simulink model "sampleModel1612"  (R2023a)
settings: Solver=VariableStepAuto  StartTime=0.0  StopTime=10.0  RelTol=1e-3
libraries: hdlsllib x6, simulink x2
settings Model: Creator=user1  LastModifiedBy=user1

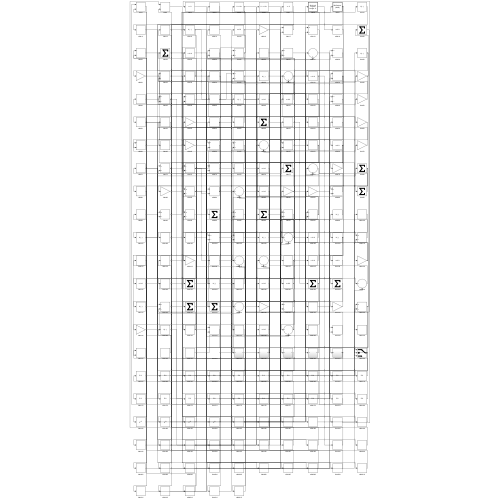
[thumbnail: Simulink's stored preview of the top-level diagram]
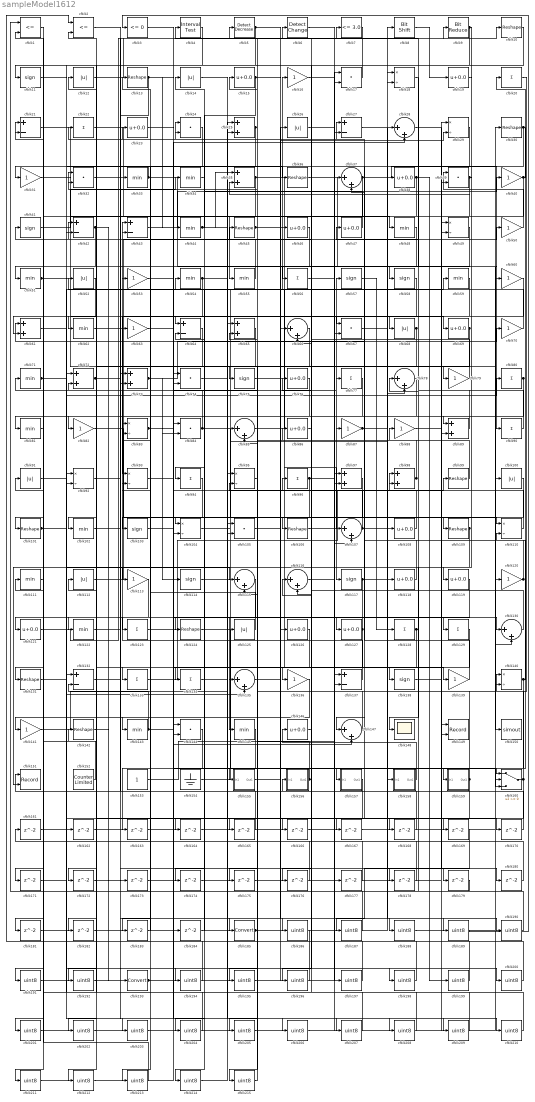
== system sampleModel1612 ==
  cfblk1 : RelationalOperator  Operator=<=  OutDataTypeStr=boolean  InputSameDT=off
  cfblk{10,13,30,36,45,99,101,106,109,124,131,142} (12 alike) : Reshape
  cfblk{12,14,26,52,68,91,100,112,125} (9 alike) : Abs  SaturateOnIntegerOverflow=off
  cfblk{33..34,44,48,51,54..55,59,62,71,81,102,111,122,143,145} (16 alike) : MinMax
  cfblk{11,41,57..58,75,103,114,117,138} (9 alike) : Signum
  cfblk{18,29,49,83,92..93,95,104,110,140} (10 alike) : Product  Inputs=*/  RndMeth=Zero  SaturateOnIntegerOverflow=on
  cfblk{17,24,32,39,67,74,84,105,144} (9 alike) : DotProduct  OutDataTypeStr=Inherit: Inherit via internal rule
  cfblk{28,37,66,78,85,107,115..116,130,135,147} (11 alike) : Sum  Inputs=|++
  cfblk{15,19,23,38,46..47,69,76,86,108,118..119,121,126..127,146} (16 alike) : Bias  Bias=0.0  SaturateOnIntegerOverflow=off
  cfblk{16,31,40,50,53,60,63,70,79,82,87..88,113,120,136,139,141} (17 alike) : Gain
  cfblk{20,22,56,77,80,90,94,96,123,128..129,133..134} (13 alike) : Sum  Inputs=+
  cfblk{21,27,42..43,64,132,137} (7 alike) : Sum  Inputs=+-
  cfblk148 : Scope
  cfblk149 : Record  FileSettingsInternal="{\"entries\":[{\"content\":{\"excelSettings\":{\"content\":{},\"type\":\"Streamout.ExcelSettings\"}},\"type\":\"Streamout.FileSettingStorage\",\"uuid\":\"\"}],\"packageUris\":[\"http:\\/\\/schema.mathworks.com\\/mf0\\/streamout_blocks\\/R2020a\"],\"version\":\"1.0\"}"  Layout=[1 1]  SignalsInternal="{\"entries\":[{\"content\":{\"signals\":[{\"content\":{\"blockPath\":[],\"dimensions\":[1],\"domain\":\"\",\"lineColor\":\"#a2142f\",\"plots\":[1],\"port\":1,\"signalID\":2323,\"signalName\":\"XY Graph:1\"},\"type\":\"RecordBlkView.Signal\",\"uuid\":\"\"},{\"content\":{\"blockPath\":[],\"dimensions\":[1],\"domain\":\"\",\"lineColor\":\"#139fff\",\"plots\":[1],\"port\":2,\"signalID\":2326,\"signalName\":\"XY Graph:2\"},\"type\":\"RecordBlkView.Signal\",\"uuid\":\"\"}]},\"type\":\"RecordBlkView.InputSignals\",\"uuid\":\"\"}],\"packageUris\":[\"http:\\/\\/schema.mathworks.com\\/mf0\\/streamout_blocks\\/R2020a\"],\"version\":\"1.0\"}"  VisualizationBindings="{\"xyplotplugin\":{\"info\":[{\"series\":[{\"bindingParametersList\":[{\"parameter\":\"X-Axis\",\"signalID\":2323,\"signalName\":\"XY Graph:1\"},{\"parameter\":\"Y-Axis\",\"signalID\":2326,\"signalName\":\"XY Graph:2\"}],\"seriesID\":49323}],\"subplotID\":1}]}}"  CompatibilityTag=XY  st=-1
  cfblk150 : ToWorkspace  VariableName=simout  SaveFormat=Timeseries  SampleTime=-1
  cfblk151 : Record  FileSettingsInternal="{\"entries\":[{\"content\":{\"excelSettings\":{\"content\":{},\"type\":\"Streamout.ExcelSettings\"}},\"type\":\"Streamout.FileSettingStorage\",\"uuid\":\"\"}],\"packageUris\":[\"http:\\/\\/schema.mathworks.com\\/mf0\\/streamout_blocks\\/R2020a\"],\"version\":\"1.0\"}"  Layout=[1 1]  SignalsInternal="{\"entries\":[{\"content\":{\"signals\":[{\"content\":{\"blockPath\":[],\"dimensions\":[1],\"domain\":\"\",\"lineColor\":\"#a2142f\",\"plots\":[1],\"port\":1,\"signalID\":2331,\"signalName\":\"XY Graph:1\"},\"type\":\"RecordBlkView.Signal\",\"uuid\":\"\"},{\"content\":{\"blockPath\":[],\"dimensions\":[1],\"domain\":\"\",\"lineColor\":\"#139fff\",\"plots\":[1],\"port\":2,\"signalID\":2334,\"signalName\":\"XY Graph:2\"},\"type\":\"RecordBlkView.Signal\",\"uuid\":\"\"}]},\"type\":\"RecordBlkView.InputSignals\",\"uuid\":\"\"}],\"packageUris\":[\"http:\\/\\/schema.mathworks.com\\/mf0\\/streamout_blocks\\/R2020a\"],\"version\":\"1.0\"}"  VisualizationBindings="{\"xyplotplugin\":{\"info\":[{\"series\":[{\"bindingParametersList\":[{\"parameter\":\"X-Axis\",\"signalID\":2331,\"signalName\":\"XY Graph:1\"},{\"parameter\":\"Y-Axis\",\"signalID\":2334,\"signalName\":\"XY Graph:2\"}],\"seriesID\":48579}],\"subplotID\":1}]}}"  CompatibilityTag=XY  st=-1
  cfblk152 : hdlsllib/Sources/Counter Limited  uplimit=7  tsamp=-1
  cfblk153 : Constant  SampleTime=-1
  cfblk154 : Ground
  cfblk155 : Subsystem
      settings: LibrarySourceBlock=|
      | hdlsllib/Ports &
      | Subsystems/Subsystem
  cfblk156 : Subsystem
      settings: LibrarySourceBlock=|
      | hdlsllib/Ports &
      | Subsystems/Subsystem
  cfblk157 : Subsystem
      settings: LibrarySourceBlock=|
      | hdlsllib/Ports &
      | Subsystems/Subsystem
  cfblk158 : Subsystem
      settings: LibrarySourceBlock=|
      | hdlsllib/Ports &
      | Subsystems/Subsystem
  cfblk159 : Subsystem
      settings: LibrarySourceBlock=|
      | hdlsllib/Ports &
      | Subsystems/Subsystem
  cfblk160 : Switch  SaturateOnIntegerOverflow=off  InputSameDT=off
  cfblk{161..184} (24 alike) : Delay  SampleTime=1
  cfblk185 : DataTypeConversion  SaturateOnIntegerOverflow=off  RndMeth=Floor
  cfblk{186..192,194..215} (29 alike) : DataTypeConversion  OutDataTypeStr=uint8  SaturateOnIntegerOverflow=off  RndMeth=Floor
  cfblk193 : DataTypeConversion  SaturateOnIntegerOverflow=off  RndMeth=Floor
  cfblk2 : RelationalOperator  Operator=<=  OutDataTypeStr=boolean  InputSameDT=off
  cfblk{25,35,61,65,72..73,89,97..98} (9 alike) : Sum
  cfblk3 : hdlsllib/Logic and Bit Operations/Compare To Zero  relop=<=  OutDataTypeStr=boolean
  cfblk4 : hdlsllib/Logic and Bit Operations/Interval Test  IntervalClosedRight=on  uplimit=0.5  IntervalClosedLeft=on  lowlimit=-0.5  OutDataTypeStr=boolean
  cfblk5 : simulink/Logic and Bit Operations/Detect Decrease  vinit=0.0  OutDataTypeStr=boolean
      settings: LibrarySourceBlock=|
      | hdlsllib/Logic and Bit
      | Operations/Detect
      | Decrease
  cfblk6 : simulink/Logic and Bit Operations/Detect Change  vinit=0  OutDataTypeStr=boolean
      settings: LibrarySourceBlock=|
      | hdlsllib/Logic and Bit
      | Operations/Detect
      | Change
  cfblk7 : hdlsllib/Logic and Bit Operations/Compare To Constant  relop=<=  const=3.0  OutDataTypeStr=boolean
  cfblk8 : hdlsllib/Logic and Bit Operations/Bit Shift  mode=Shift Left Logical  N=0
  cfblk9 : hdlsllib/Logic and Bit Operations/Bit Reduce  mode=AND
  wires:
  cfblk137/1 -> cfblk43/1
  cfblk57/1 -> cfblk128/1
  cfblk121/1 -> cfblk7/1
  cfblk5/1 -> cfblk42/2, cfblk178/1
  cfblk39/1 -> cfblk55/1, cfblk109/1, cfblk35/2
  cfblk112/1 -> cfblk45/1
  cfblk98/1 -> cfblk53/1, cfblk32/1
  cfblk114/1 -> cfblk16/1
  cfblk75/1 -> cfblk139/1
  cfblk37/1 -> cfblk90/1, cfblk66/2
  cfblk107/1 -> cfblk96/1, cfblk160/3
  cfblk130/1 -> cfblk41/1
  cfblk106/1 -> cfblk57/1
  cfblk62/1 -> cfblk25/1
  cfblk35/1 -> cfblk117/1, cfblk124/1
  cfblk113/1 -> cfblk121/1
  cfblk82/1 -> cfblk110/1
  cfblk31/1 -> cfblk68/1
  cfblk143/1 -> cfblk12/1, cfblk99/1
  cfblk158/1(Out1) -> cfblk146/1
  cfblk8/1 -> cfblk19/1
  cfblk36/1 -> cfblk120/1
  cfblk131/1 -> cfblk59/1
  cfblk99/1 -> cfblk78/1
  cfblk12/1 -> cfblk9/1
  cfblk51/1 -> cfblk150/1, cfblk191/1, cfblk194/1
  cfblk154/1 -> cfblk98/1
  cfblk33/1 -> cfblk158/1(In1), cfblk31/1
  cfblk10/1 -> cfblk56/1
  cfblk139/1 -> cfblk27/1
  cfblk64/1 -> cfblk93/1
  cfblk46/1 -> cfblk133/1
  cfblk1/1 -> cfblk51/1
  cfblk25/1 -> cfblk5/1, cfblk202/1
  cfblk125/1 -> cfblk13/1
  cfblk66/1 -> cfblk82/1
  cfblk84/1 -> cfblk106/1, cfblk72/2
  cfblk109/1 -> cfblk148/1, cfblk151/2
  cfblk53/1 -> cfblk155/1(In1)
  cfblk153/1 -> cfblk27/2
  cfblk73/1 -> cfblk70/1, cfblk84/2, cfblk28/2, cfblk138/1
  cfblk140/1 -> cfblk110/2, cfblk183/1
  cfblk118/1 -> cfblk61/1
  cfblk50/1 -> cfblk39/1
  cfblk9/1 -> cfblk119/1, cfblk92/2
  cfblk15/1 -> cfblk104/1, cfblk79/1
  cfblk38/1 -> cfblk176/1, cfblk199/1
  cfblk68/1 -> cfblk136/1, cfblk75/1
  cfblk11/1 -> cfblk36/1
  cfblk133/1 -> cfblk8/1
  cfblk22/1 -> cfblk118/1
  cfblk142/1 -> cfblk193/1
  cfblk56/1 -> cfblk137/2
  cfblk67/1 -> cfblk78/2
  cfblk2/1 -> cfblk185/1
  cfblk123/1 -> cfblk28/1
  cfblk42/1 -> cfblk101/1, cfblk173/1
  cfblk87/1 -> cfblk129/1, cfblk37/2
  cfblk117/1 -> cfblk127/1, cfblk160/2, cfblk181/1
  cfblk79/1 -> cfblk24/1
  cfblk104/1 -> cfblk18/1
  cfblk141/1 -> cfblk25/2
  cfblk41/1 -> cfblk34/1
  cfblk55/1 -> cfblk21/1
  cfblk111/1 -> cfblk131/1
  cfblk90/1 -> cfblk47/1
  cfblk135/1 -> cfblk46/1
  cfblk76/1 -> cfblk134/1
  cfblk136/1 -> cfblk141/1
  cfblk80/1 -> cfblk81/1, cfblk149/2
  cfblk100/1 -> cfblk147/1
  cfblk7/1 -> cfblk62/1
  cfblk44/1 -> cfblk24/2, cfblk67/1, cfblk35/1
  cfblk20/1 -> cfblk140/1
  cfblk24/1 -> cfblk123/1
  cfblk19/1 -> cfblk89/1
  cfblk43/1 -> cfblk40/1
  cfblk52/1 -> cfblk61/2
  cfblk58/1 -> cfblk83/1
  cfblk160/1 -> cfblk42/1, cfblk174/1, cfblk175/1
  cfblk23/1 -> cfblk130/1
  cfblk21/1 -> cfblk84/1
  cfblk72/1 -> cfblk33/1, cfblk212/1
  cfblk110/1 -> cfblk15/1
  cfblk124/1 -> cfblk157/1(In1)
  cfblk48/1 -> cfblk102/1
  cfblk127/1 -> cfblk122/1, cfblk192/1
  cfblk96/1 -> cfblk103/1, cfblk159/1(In1)
  cfblk47/1 -> cfblk14/1
  cfblk30/1 -> cfblk160/1, cfblk144/2
  cfblk61/1 -> cfblk115/1
  cfblk26/1 -> cfblk60/1
  cfblk60/1 -> cfblk64/1
  cfblk101/1 -> cfblk80/1, cfblk135/2
  cfblk138/1 -> cfblk149/1
  cfblk85/1 -> cfblk17/2
  cfblk70/1 -> cfblk23/1
  cfblk59/1 -> cfblk113/1
  cfblk103/1 -> cfblk77/1
  cfblk45/1 -> cfblk29/2, cfblk168/1
  cfblk89/1 -> cfblk4/1
  cfblk40/1 -> cfblk20/1, cfblk211/1
  cfblk159/1(Out1) -> cfblk151/1, cfblk71/1, cfblk169/1
  cfblk156/1(Out1) -> cfblk85/2, cfblk86/1
  cfblk94/1 -> cfblk143/1
  cfblk147/1 -> cfblk52/1, cfblk32/2
  cfblk120/1 -> cfblk87/1, cfblk22/1
  cfblk83/1 -> cfblk50/1, cfblk114/1
  cfblk17/1 -> cfblk11/1
  cfblk71/1 -> cfblk170/1, cfblk203/1
  cfblk108/1 -> cfblk76/1
  cfblk115/1 -> cfblk145/1
  cfblk92/1 -> cfblk10/1
  cfblk69/1 -> cfblk104/2, cfblk135/1
  cfblk28/1 -> cfblk89/2
  cfblk155/1(Out1) -> cfblk126/1
  cfblk34/1 -> cfblk94/1
  cfblk128/1 -> cfblk98/2, cfblk164/1
  cfblk14/1 -> cfblk125/1
  cfblk146/1 -> cfblk6/1
  cfblk152/1 -> cfblk111/1
  cfblk29/1 -> cfblk107/1
  cfblk18/1 -> cfblk58/1
  cfblk54/1 -> cfblk69/1, cfblk63/1
  cfblk16/1 -> cfblk48/1
  cfblk13/1 -> cfblk73/2, cfblk147/2, cfblk44/1
  cfblk77/1 -> cfblk115/2
  cfblk161/1 -> cfblk85/1
  cfblk91/1 -> cfblk162/1
  cfblk162/1 -> cfblk17/1
  cfblk144/1 -> cfblk163/1
  cfblk164/1 -> cfblk64/2
  cfblk126/1 -> cfblk165/1
  cfblk165/1 -> cfblk21/2
  cfblk134/1 -> cfblk166/1
  cfblk166/1 -> cfblk140/2
  cfblk78/1 -> cfblk167/1
  cfblk167/1 -> cfblk130/2
  cfblk168/1 -> cfblk83/2
  cfblk170/1 -> cfblk73/1
  cfblk81/1 -> cfblk171/1
  cfblk171/1 -> cfblk92/1
  cfblk4/1 -> cfblk172/1
  cfblk173/1 -> cfblk39/2
  cfblk174/1 -> cfblk29/1
  cfblk175/1 -> cfblk107/2
  cfblk176/1 -> cfblk1/2
  cfblk177/1 -> cfblk43/2
  cfblk178/1 -> cfblk72/1
  cfblk122/1 -> cfblk179/1
  cfblk179/1 -> cfblk1/1
  cfblk88/1 -> cfblk180/1
  cfblk180/1 -> cfblk137/1
  cfblk181/1 -> cfblk18/2
  cfblk157/1(Out1) -> cfblk182/1
  cfblk182/1 -> cfblk37/1
  cfblk183/1 -> cfblk93/2
  cfblk63/1 -> cfblk184/1
  cfblk184/1 -> cfblk54/1
  cfblk185/1 -> cfblk38/1, cfblk67/2, cfblk108/1
  cfblk32/1 -> cfblk186/1
  cfblk186/1 -> cfblk2/1
  cfblk169/1 -> cfblk187/1
  cfblk187/1 -> cfblk2/2
  cfblk3/1 -> cfblk188/1
  cfblk188/1 -> cfblk100/1
  cfblk27/1 -> cfblk189/1
  cfblk189/1 -> cfblk3/1
  cfblk105/1 -> cfblk190/1
  cfblk190/1 -> cfblk88/1
  cfblk191/1 -> cfblk105/1
  cfblk192/1 -> cfblk105/2
  cfblk193/1 -> cfblk66/1, cfblk26/1
  cfblk194/1 -> cfblk142/1
  cfblk95/1 -> cfblk195/1
  cfblk195/1 -> cfblk177/1
  cfblk86/1 -> cfblk196/1
  cfblk196/1 -> cfblk95/1
  cfblk6/1 -> cfblk197/1
  cfblk197/1 -> cfblk95/2
  cfblk116/1 -> cfblk198/1
  cfblk198/1 -> cfblk112/1
  cfblk199/1 -> cfblk116/1
  cfblk172/1 -> cfblk200/1
  cfblk200/1 -> cfblk116/2
  cfblk49/1 -> cfblk201/1
  cfblk201/1 -> cfblk30/1
  cfblk202/1 -> cfblk49/1
  cfblk203/1 -> cfblk49/2
  cfblk97/1 -> cfblk204/1
  cfblk204/1 -> cfblk161/1
  cfblk129/1 -> cfblk205/1
  cfblk205/1 -> cfblk97/1
  cfblk102/1 -> cfblk206/1
  cfblk206/1 -> cfblk97/2
  cfblk132/1 -> cfblk207/1
  cfblk207/1 -> cfblk156/1(In1)
  cfblk163/1 -> cfblk208/1
  cfblk208/1 -> cfblk132/1
  cfblk93/1 -> cfblk209/1
  cfblk209/1 -> cfblk132/2
  cfblk74/1 -> cfblk210/1
  cfblk210/1 -> cfblk144/1
  cfblk211/1 -> cfblk74/1
  cfblk212/1 -> cfblk74/2
  cfblk65/1 -> cfblk213/1
  cfblk213/1 -> cfblk91/1
  cfblk145/1 -> cfblk214/1
  cfblk214/1 -> cfblk65/1
  cfblk119/1 -> cfblk215/1
  cfblk215/1 -> cfblk65/2

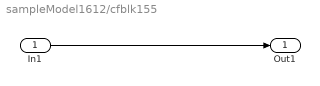
== system sampleModel1612/cfblk155 ==
  In1 : Inport
  Out1 : Outport
  wires:
  In1/1 -> Out1/1

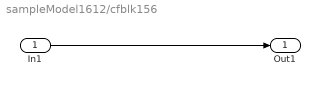
== system sampleModel1612/cfblk156 ==
  In1 : Inport
  Out1 : Outport
  wires:
  In1/1 -> Out1/1

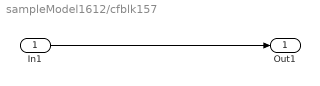
== system sampleModel1612/cfblk157 ==
  In1 : Inport
  Out1 : Outport
  wires:
  In1/1 -> Out1/1

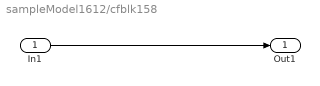
== system sampleModel1612/cfblk158 ==
  In1 : Inport
  Out1 : Outport
  wires:
  In1/1 -> Out1/1

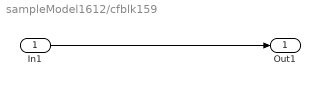
== system sampleModel1612/cfblk159 ==
  In1 : Inport
  Out1 : Outport
  wires:
  In1/1 -> Out1/1
